simulink model "nonLinearModel2"  (R2014b)
settings: Solver=ode3  StartTime=0.0  StopTime=TIME_SIM  FixedStep=STEP_SIZE  RelTol=1e-3
values from neighbouring files (symbols this model uses):
  b1 = 2.6826    [main.m]    (also in mainbis.m)
  b2 = -4.0269*10^3    (= -4026.9)    [main.m]    (also in mainbis.m)
  Bl0 = 14.54    [main.m]    (also in mainbis.m)
  k0 = 6259.3    [main.m]    (also in mainbis.m)
  k1 = -1.4562*10^5    (= -145620)    [main.m]    (also in mainbis.m)
  k2 = 2.6106*10^7    (= 26106000)    [main.m]    (also in mainbis.m)
  l1 = -5.2937*10^(-1)    (= -0.52937)    [main.m]    (also in mainbis.m)
  l2 = -1.2012*10^2    (= -120.12)    [main.m]    (also in mainbis.m)
  Le0 = 5.65*10^(-3)    (= 0.00565)    [main.m]    (also in mainbis.m)
  mt = 52.08*10^(-3)    (= 0.05208)    [main.m]    (also in mainbis.m)
  Re = 7.9    [main.m]    (also in mainbis.m)
  Rm = 2.628    [main.m]    (also in mainbis.m)
settings Model: Creator=s150810  LastModifiedBy=Kate
settings DataIOCC: SaveState=on

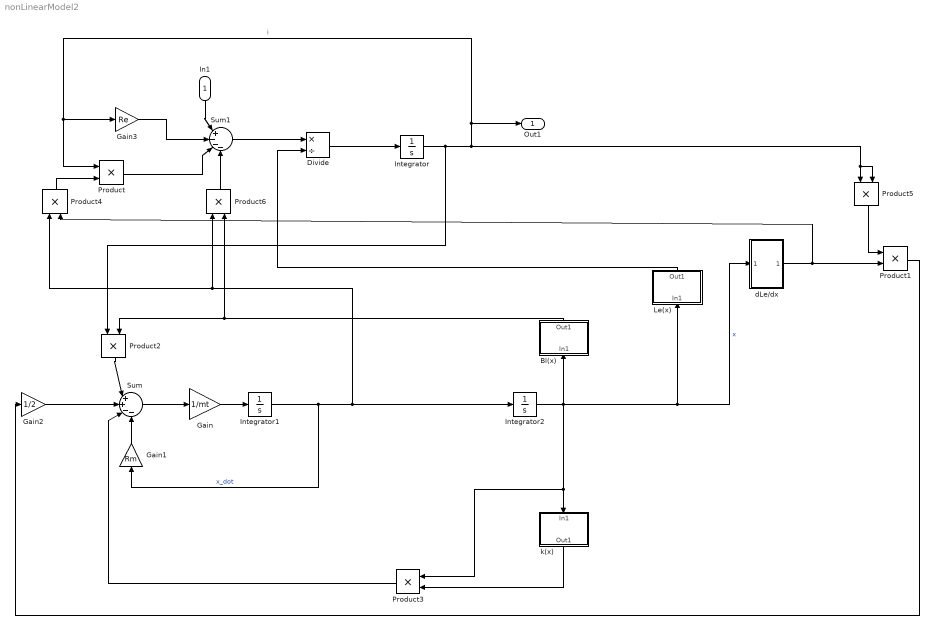
== system nonLinearModel2 ==
  In1 : Inport
  Bl(x) : Subsystem
  Divide : Product  Inputs=*/
  Gain : Gain  Gain=1/mt
  Gain1 : Gain  Gain=Rm
  Gain2 : Gain  Gain=1/2
  Gain3 : Gain  Gain=Re
  Integrator : Integrator  Priority=3
  Integrator1 : Integrator  Priority=2
  Integrator2 : Integrator  Priority=1
  Le(x) : Subsystem
  Product{,1..6} (7 alike) : Product
  Sum : Sum  Inputs=|++--
  Sum1 : Sum  Inputs=|+---
  dLe/dx : Subsystem
  k(x) : Subsystem
  Out1 : Outport
  wires:
  Integrator1/1 -> Gain1/1, Product6/1, Product4/1, Integrator2/1  "x_dot"
  Integrator2/1 -> Product3/1, k(x)/1(In1), Bl(x)/1(In1), Le(x)/1(In1), dLe/dx/1(In1)  "x"
  Integrator/1 -> Product2/1, Out1/1, Product/1, Gain3/1, Product5/1, Product5/2  "i"
  Gain/1 -> Integrator1/1
  Sum/1 -> Gain/1
  Product2/1 -> Sum/1
  Bl(x)/1(Out1) -> Product6/2, Product2/2
  Gain1/1 -> Sum/4
  k(x)/1(Out1) -> Product3/2
  Product3/1 -> Sum/3
  Gain2/1 -> Sum/2
  Product1/1 -> Gain2/1
  Product5/1 -> Product1/1
  dLe/dx/1(Out1) -> Product1/2, Product4/2
  Divide/1 -> Integrator/1
  Le(x)/1(Out1) -> Divide/2
  Sum1/1 -> Divide/1
  In1/1 -> Sum1/1
  Gain3/1 -> Sum1/2
  Product4/1 -> Product/2
  Product/1 -> Sum1/3
  Product6/1 -> Sum1/4

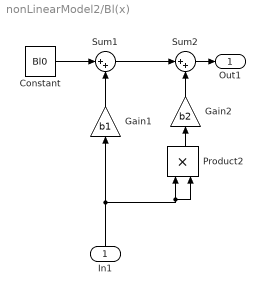
== system nonLinearModel2/Bl(x) ==
  In1 : Inport
  Constant : Constant  Value=Bl0
  Gain1 : Gain  Gain=b1
  Gain2 : Gain  Gain=b2
  Product2 : Product
  Sum1 : Sum  Inputs=|++
  Sum2 : Sum  Inputs=|++
  Out1 : Outport
  wires:
  Gain2/1 -> Sum2/2
  Product2/1 -> Gain2/1
  Constant/1 -> Sum1/1
  Sum1/1 -> Sum2/1
  In1/1 -> Product2/2, Product2/1, Gain1/1
  Sum2/1 -> Out1/1
  Gain1/1 -> Sum1/2

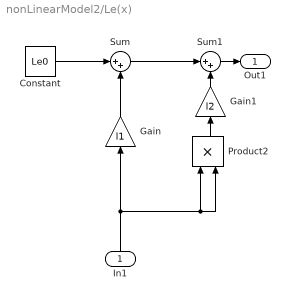
== system nonLinearModel2/Le(x) ==
  In1 : Inport
  Constant : Constant  Value=Le0
  Gain : Gain  Gain=l1
  Gain1 : Gain  Gain=l2
  Product2 : Product
  Sum : Sum  Inputs=|++
  Sum1 : Sum  Inputs=|++
  Out1 : Outport
  wires:
  Sum1/1 -> Out1/1
  In1/1 -> Gain/1, Product2/1, Product2/2
  Product2/1 -> Gain1/1
  Constant/1 -> Sum/1
  Gain1/1 -> Sum1/2
  Gain/1 -> Sum/2
  Sum/1 -> Sum1/1

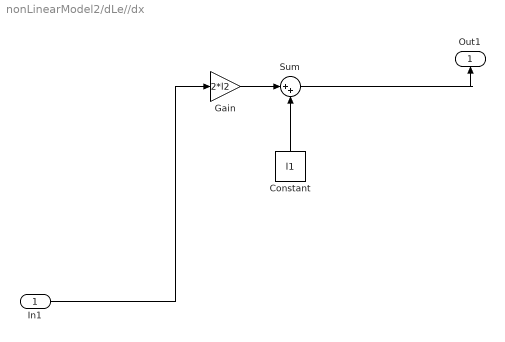
== system nonLinearModel2/dLe//dx ==
  In1 : Inport
  Constant : Constant  Value=l1
  Gain : Gain  Gain=2*l2
  Sum : Sum  Inputs=|++
  Out1 : Outport
  wires:
  Sum/1 -> Out1/1
  Constant/1 -> Sum/2
  Gain/1 -> Sum/1
  In1/1 -> Gain/1

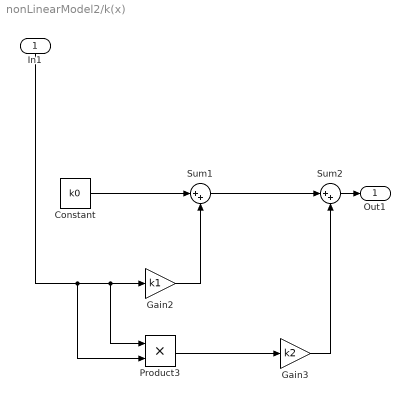
== system nonLinearModel2/k(x) ==
  In1 : Inport
  Constant : Constant  Value=k0
  Gain2 : Gain  Gain=k1
  Gain3 : Gain  Gain=k2
  Product3 : Product
  Sum1 : Sum  Inputs=|++
  Sum2 : Sum  Inputs=|++
  Out1 : Outport
  wires:
  In1/1 -> Product3/2, Product3/1, Gain2/1
  Sum2/1 -> Out1/1
  Gain2/1 -> Sum1/2
  Constant/1 -> Sum1/1
  Gain3/1 -> Sum2/2
  Product3/1 -> Gain3/1
  Sum1/1 -> Sum2/1
